simulink model "Problem5f_Sim"  (R2015b)
settings: Solver=VariableStepAuto  StartTime=0.0  StopTime=10.0  RelTol=1e-3
libraries: simulink_extras x3
settings Model: Creator=dmartin_a  LastModifiedBy=dmartin_a

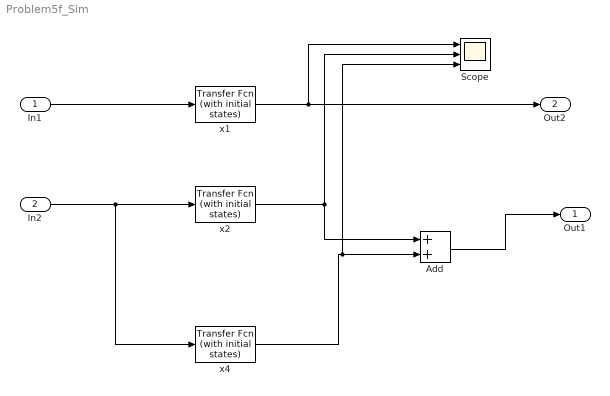
== system Problem5f_Sim ==
  In1 : Inport
  In2 : Inport  Port=2
  Add : Sum
  Scope : Scope  NumInputPorts=3
  x1 : simulink_extras/Additional Linear/Transfer Fcn (with initial states)  N=[2 4]  D=[1 4 3]  X0=1
  x2 : simulink_extras/Additional Linear/Transfer Fcn (with initial states)  N=[1]  D=[1 2 1]  X0=1
  x4 : simulink_extras/Additional Linear/Transfer Fcn (with initial states)  N=[1]  D=[1 1]  X0=1
  Out1 : Outport
  Out2 : Outport  Port=2
  wires:
  x4/1 -> Scope/3, Add/2
  x2/1 -> Add/1, Scope/2
  Add/1 -> Out1/1
  x1/1 -> Out2/1, Scope/1
  In1/1 -> x1/1
  In2/1 -> x4/1, x2/1
